simulink model "chapter_5"  (R2019b)
settings: Solver=VariableStepAuto  StartTime=0.0  StopTime=.2  RelTol=1e-3
libraries: cstblocks x6
settings Model: Creator=tomas  LastModifiedBy=lunap
settings DataIOCC: ReturnWorkspaceOutputs=off
settings DebuggingCC: ArithmeticOperatorsInVariantConditions=warning
settings SFSimCC: SimUseLocalCustomCode=off  CustomCodeUndefinedFunction=UseInterfaceOnly
settings RTWCC: RTWUseLocalCustomCode=off

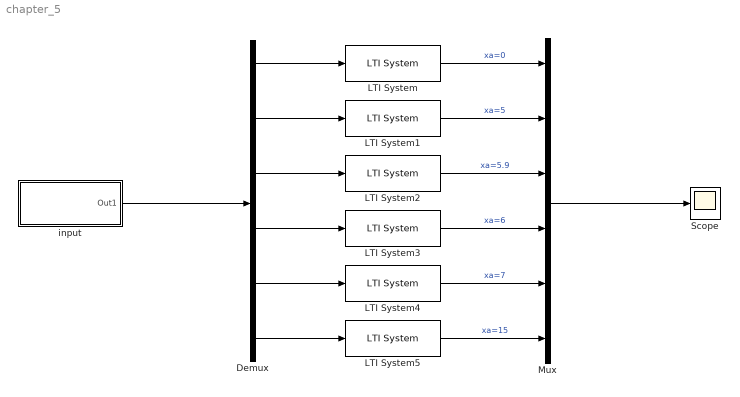
== system chapter_5 ==
  Demux : Demux  Outputs=6
  LTI System : cstblocks/LTI System  sys=G1  IC=[]
  LTI System1 : cstblocks/LTI System  sys=G2  IC=[]
  LTI System2 : cstblocks/LTI System  sys=G3  IC=[]
  LTI System3 : cstblocks/LTI System  sys=G4  IC=[]
  LTI System4 : cstblocks/LTI System  sys=G5  IC=[]
  LTI System5 : cstblocks/LTI System  sys=G6  IC=[]
  Mux : Mux  Inputs=6
  Scope : Scope
  input : Subsystem
  wires:
  Demux/1 -> LTI System/1
  Demux/2 -> LTI System1/1
  Demux/3 -> LTI System2/1
  Demux/4 -> LTI System3/1
  Demux/5 -> LTI System4/1
  LTI System1/1 -> Mux/2  "xa=5"
  LTI System/1 -> Mux/1  "xa=0"
  LTI System2/1 -> Mux/3  "xa=5.9"
  LTI System3/1 -> Mux/4  "xa=6"
  LTI System4/1 -> Mux/5  "xa=7"
  Mux/1 -> Scope/1
  Demux/6 -> LTI System5/1
  LTI System5/1 -> Mux/6  "xa=15"
  input/1(Out1) -> Demux/1

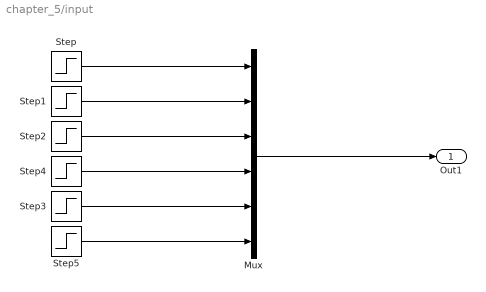
== system chapter_5/input ==
  Mux : Mux  Inputs=6
  Step{,1..5} (6 alike) : Step  Time=0  After=-1  SampleTime=0
  Out1 : Outport  VectorParamsAs1DForOutWhenUnconnected=off
  wires:
  Step/1 -> Mux/1
  Step1/1 -> Mux/2
  Step2/1 -> Mux/3
  Step4/1 -> Mux/4
  Step3/1 -> Mux/5
  Mux/1 -> Out1/1
  Step5/1 -> Mux/6
